simulink model "Downsampling"  (R2017a)
settings: Solver=VariableStepAuto  StartTime=0.0  StopTime=16  RelTol=1e-3
settings Model: Creator=Arthur  LastModifiedBy=Arthur

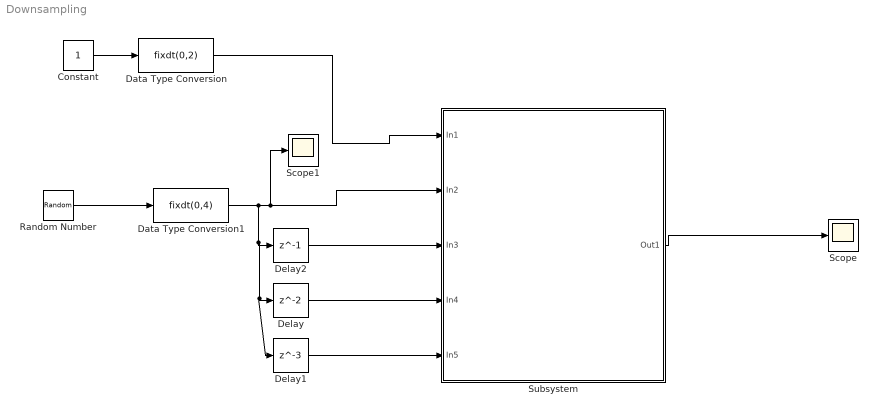
== system Downsampling ==
  Constant : Constant  OutMin=1  OutMax=1  OutDataTypeStr=fixdt(0,2)
  Data Type Conversion : DataTypeConversion  OutMin=1  OutMax=1  OutDataTypeStr=fixdt(0,2)
  Data Type Conversion1 : DataTypeConversion  OutMin=0  OutMax=8  OutDataTypeStr=fixdt(0,4)  SaturateOnIntegerOverflow=on
  Delay : Delay
  Delay1 : Delay  DelayLength=3
  Delay2 : Delay  DelayLength=1
  Random Number : RandomNumber  Variance=20  SampleTime=1
  Scope : Scope
  Scope1 : Scope
  Subsystem : Subsystem
  wires:
  Constant/1 -> Data Type Conversion/1
  Data Type Conversion/1 -> Subsystem/1(In1)
  Subsystem/1(Out1) -> Scope/1
  Random Number/1 -> Data Type Conversion1/1
  Data Type Conversion1/1 -> Delay1/1, Delay/1, Delay2/1, Scope1/1, Subsystem/2(In2)
  Delay2/1 -> Subsystem/3(In3)
  Delay/1 -> Subsystem/4(In4)
  Delay1/1 -> Subsystem/5(In5)

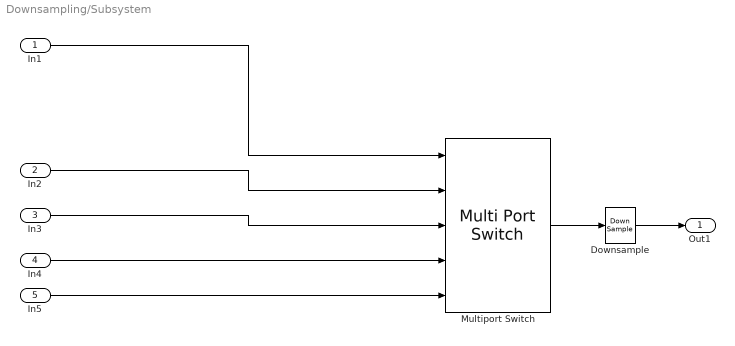
== system Downsampling/Subsystem ==
  In1 : Inport
  In2 : Inport  Port=2
  In3 : Inport  Port=3
  In4 : Inport  Port=4
  In5 : Inport  Port=5
  Downsample : DownSample  N=4
  Multiport Switch : MultiPortSwitch  Inputs=4  DataPortIndices={1,2,3,4}  OutMin=1  OutMax=4  OutDataTypeStr=fixdt(0,3)
  Out1 : Outport
  wires:
  Downsample/1 -> Out1/1
  Multiport Switch/1 -> Downsample/1
  In2/1 -> Multiport Switch/2
  In3/1 -> Multiport Switch/3
  In4/1 -> Multiport Switch/4
  In5/1 -> Multiport Switch/5
  In1/1 -> Multiport Switch/1
